simulink model "systeme_sol_2017a_PID"  (R2017a)
settings: Solver=VariableStepAuto  StartTime=0.0  StopTime=50000  RelTol=1e-3
libraries: simulink x1
settings Model: Creator=julien  LastModifiedBy=admin
settings DataIOCC: ReturnWorkspaceOutputs=on
settings SFSimCC: SimUseLocalCustomCode=on
settings RTWCC: RTWUseLocalCustomCode=on

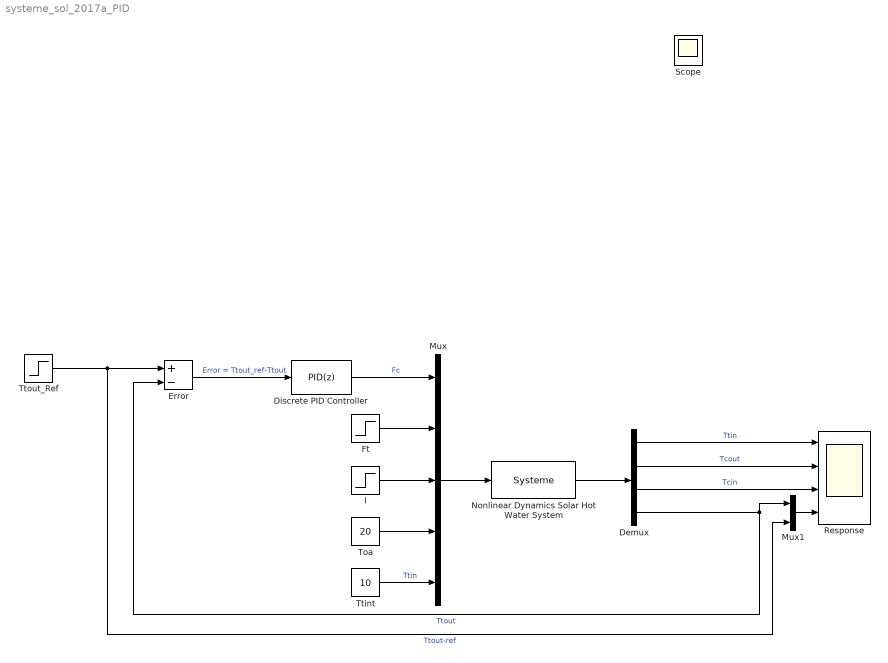
== system systeme_sol_2017a_PID ==
  Demux : Demux
  Discrete PID Controller : simulink/Continuous/PID Controller  Controller=PID  TimeDomain=Discrete-time  SampleTime=-1  IntegratorMethod=Forward Euler  FilterMethod=Forward Euler  Form=Parallel  UseFilter=on  ControllerParametersSource=internal  P=-0.005  I=0  D=0  N=100  InitialConditionSource=internal  InitialConditionForIntegrator=0  InitialConditionForFilter=0  ExternalReset=none  LimitOutput=on  UpperSaturationLimit=2.5e-5  LowerSaturationLimit=0  LinearizeAsGain=off  AntiWindupMode=none  Kb=1  TrackingMode=off  Kt=1  PParamMin=[]  PParamMax=[]  IParamMin=[]  IParamMax=[]  DParamMin=[]  DParamMax=[]  NParamMin=[]  NParamMax=[]  KbParamMin=[]  KbParamMax=[]  KtParamMin=[]  KtParamMax=[]  POutMin=[]  POutMax=[]  IOutMin=[]  IOutMax=[]  DOutMin=[]  DOutMax=[]  NOutMin=[]  NOutMax=[]  KbOutMin=[]  KbOutMax=[]  KtOutMin=[]  KtOutMax=[]  IntegratorOutMin=[]  IntegratorOutMax=[]  FilterOutMin=[]  FilterOutMax=[]  SumOutMin=[]  SumOutMax=[]  SumI1OutMin=[]  SumI1OutMax=[]  SumI2OutMin=[]  SumI2OutMax=[]  SumI3OutMin=[]  SumI3OutMax=[]  SumDOutMin=[]  SumDOutMax=[]  SaturationOutMin=[]  SaturationOutMax=[]  IntegratorContinuousStateAttributes=''  IntegratorStateMustResolveToSignalObject=off  IntegratorRTWStateStorageClass=Auto  FilterContinuousStateAttributes=''  FilterStateMustResolveToSignalObject=off  FilterRTWStateStorageClass=Auto  DifferentiatorICPrevScaledInput=0  DifferentiatorOutMin=[]  DifferentiatorOutMax=[]  InitialConditionSetting=State (most efficient)
  "Error " : Sum  Inputs=+-
  Ft : Step  Time=0  After=1e-5  SampleTime=0
  I : Step  Time=50000  Before=1000  After=1000  SampleTime=0
  Mux : Mux  Inputs=5
  Mux1 : Mux  Inputs=2
  Nonlinear Dynamics Solar Hot Water System : S-Function  FunctionName=Systeme  Parameters=60,27.5,47.5  SFunctionDeploymentMode=off  EnableBusSupport=off
  "Response " : Scope  NumInputPorts=4
  Toa : Constant  Value=20
  Ttint : Constant  Value=10
  "Ttout_Ref " : Step  Time=20000  Before=52.5  After=47.5  SampleTime=0
  Scope : Scope
  wires:
  Discrete PID Controller/1 -> Mux/1  "Fc"
  Ft/1 -> Mux/2
  I/1 -> Mux/3
  Toa/1 -> Mux/4
  Ttint/1 -> Mux/5  "Ttin"
  Mux/1 -> Nonlinear Dynamics Solar Hot Water System/1
  Nonlinear Dynamics Solar Hot Water System/1 -> Demux/1
  Demux/4 -> Mux1/1, "Error "/2  "Ttout"
  Demux/3 -> "Response "/3  "Tcin"
  Demux/2 -> "Response "/2  "Tcout"
  Demux/1 -> "Response "/1  "Ttin"
  "Error "/1 -> Discrete PID Controller/1  "Error = Ttout_ref-Ttout"
  "Ttout_Ref "/1 -> Mux1/2, "Error "/1  "Ttout-ref"
  Mux1/1 -> "Response "/4
